simulink model "massbalancer"  (R2024a)
settings: Solver=VariableStepAuto  StartTime=0.0  StopTime=inf  RelTol=1e-3
libraries: matrix_library x36, sharedutil x2, sharedtransform x2, dspinverses x1, aerolibutil x1
(part 2 of 3)

== system massbalancer/Wdot b/I_r/Subsystem3 ==
  In1 : Inport
  Reshape : Reshape  OutputDimensionality=Column vector (2-D)  OutputDimensions=[1,3]
  Selector : Selector  InputPortWidth=9  IndexOptions=Index vector (dialog)  Indices=[1]  OutputSizes=1
  Selector1 : Selector  InputPortWidth=9  IndexOptions=Index vector (dialog)  Indices=[2]  OutputSizes=1
  Selector2 : Selector  InputPortWidth=9  IndexOptions=Index vector (dialog)  Indices=[3]  OutputSizes=1
  Selector3 : Selector  InputPortWidth=9  IndexOptions=Index vector (dialog)  Indices=[4]  OutputSizes=1
  Selector4 : Selector  InputPortWidth=9  IndexOptions=Index vector (dialog)  Indices=[5]  OutputSizes=1
  Selector5 : Selector  InputPortWidth=9  IndexOptions=Index vector (dialog)  Indices=[6]  OutputSizes=1
  Selector6 : Selector  InputPortWidth=9  IndexOptions=Index vector (dialog)  Indices=[7]  OutputSizes=1
  Selector7 : Selector  InputPortWidth=9  IndexOptions=Index vector (dialog)  Indices=[8]  OutputSizes=1
  Selector8 : Selector  InputPortWidth=9  IndexOptions=Index vector (dialog)  Indices=[9]  OutputSizes=1
  Vector Concatenate : Concatenate  NumInputs=3  Mode=Multidimensional array
  Vector Concatenate1 : Concatenate  NumInputs=3  Mode=Multidimensional array
  Vector Concatenate2 : Concatenate  NumInputs=3  Mode=Multidimensional array
  Out1 : Outport
  Out2 : Outport  Port=2
  Out3 : Outport  Port=3
  wires:
  Selector2/1 -> Vector Concatenate/3
  Vector Concatenate/1 -> Out1/1
  Selector8/1 -> Vector Concatenate2/3
  Selector4/1 -> Vector Concatenate1/2
  Selector6/1 -> Vector Concatenate2/1
  In1/1 -> Reshape/1
  Reshape/1 -> Selector8/1, Selector7/1, Selector6/1, Selector5/1, Selector4/1, Selector3/1, Selector2/1, Selector1/1, Selector/1
  Selector/1 -> Vector Concatenate/1
  Selector5/1 -> Vector Concatenate1/3
  Selector7/1 -> Vector Concatenate2/2
  Vector Concatenate2/1 -> Out3/1
  Vector Concatenate1/1 -> Out2/1
  Selector1/1 -> Vector Concatenate/2
  Selector3/1 -> Vector Concatenate1/1

== system massbalancer/Wdot b/I_r/Subsystem4 ==
  In1 : Inport
  Reshape : Reshape  OutputDimensionality=Column vector (2-D)  OutputDimensions=[1,3]
  Selector : Selector  InputPortWidth=9  IndexOptions=Index vector (dialog)  Indices=[1]  OutputSizes=1
  Selector1 : Selector  InputPortWidth=9  IndexOptions=Index vector (dialog)  Indices=[2]  OutputSizes=1
  Selector2 : Selector  InputPortWidth=9  IndexOptions=Index vector (dialog)  Indices=[3]  OutputSizes=1
  Selector3 : Selector  InputPortWidth=9  IndexOptions=Index vector (dialog)  Indices=[4]  OutputSizes=1
  Selector4 : Selector  InputPortWidth=9  IndexOptions=Index vector (dialog)  Indices=[5]  OutputSizes=1
  Selector5 : Selector  InputPortWidth=9  IndexOptions=Index vector (dialog)  Indices=[6]  OutputSizes=1
  Selector6 : Selector  InputPortWidth=9  IndexOptions=Index vector (dialog)  Indices=[7]  OutputSizes=1
  Selector7 : Selector  InputPortWidth=9  IndexOptions=Index vector (dialog)  Indices=[8]  OutputSizes=1
  Selector8 : Selector  InputPortWidth=9  IndexOptions=Index vector (dialog)  Indices=[9]  OutputSizes=1
  Vector Concatenate : Concatenate  NumInputs=3  Mode=Multidimensional array
  Vector Concatenate1 : Concatenate  NumInputs=3  Mode=Multidimensional array
  Vector Concatenate2 : Concatenate  NumInputs=3  Mode=Multidimensional array
  Out1 : Outport
  Out2 : Outport  Port=2
  Out3 : Outport  Port=3
  wires:
  Selector3/1 -> Vector Concatenate1/1
  Selector1/1 -> Vector Concatenate/2
  Vector Concatenate1/1 -> Out2/1
  Vector Concatenate2/1 -> Out3/1
  Selector7/1 -> Vector Concatenate2/2
  Selector5/1 -> Vector Concatenate1/3
  Selector/1 -> Vector Concatenate/1
  Reshape/1 -> Selector/1, Selector1/1, Selector2/1, Selector3/1, Selector4/1, Selector5/1, Selector6/1, Selector7/1, Selector8/1
  In1/1 -> Reshape/1
  Selector6/1 -> Vector Concatenate2/1
  Selector4/1 -> Vector Concatenate1/2
  Selector8/1 -> Vector Concatenate2/3
  Vector Concatenate/1 -> Out1/1
  Selector2/1 -> Vector Concatenate/3

== system massbalancer/Subsystem1/Subsystem1/Subsystem/Enabled Subsystem ==
  In1 : Inport
  Enable : EnablePort
  Out1 : Outport
  wires:
  In1/1 -> Out1/1

== system massbalancer/Subsystem1/Subsystem1/Subsystem1/Enabled Subsystem ==
  In1 : Inport
  Enable : EnablePort
  Out1 : Outport
  wires:
  In1/1 -> Out1/1

== system massbalancer/Subsystem1/Subsystem1/Subsystem2/Enabled Subsystem ==
  In1 : Inport
  Enable : EnablePort
  Out1 : Outport
  wires:
  In1/1 -> Out1/1

== system massbalancer/Subsystem1/Subsystem2/Subsystem/Enabled Subsystem ==
  In1 : Inport
  Enable : EnablePort
  Out1 : Outport
  wires:
  In1/1 -> Out1/1

== system massbalancer/Subsystem1/Subsystem2/Subsystem1/Enabled Subsystem ==
  In1 : Inport
  Enable : EnablePort
  Out1 : Outport
  wires:
  In1/1 -> Out1/1

== system massbalancer/Subsystem1/Subsystem2/Subsystem2/Enabled Subsystem ==
  In1 : Inport
  Enable : EnablePort
  Out1 : Outport
  wires:
  In1/1 -> Out1/1

== system massbalancer/Subsystem1/Subsystem3/Subsystem/Enabled Subsystem ==
  In1 : Inport
  Enable : EnablePort
  Out1 : Outport
  wires:
  In1/1 -> Out1/1

== system massbalancer/Subsystem1/Subsystem3/Subsystem1/Enabled Subsystem ==
  In1 : Inport
  Enable : EnablePort
  Out1 : Outport
  wires:
  In1/1 -> Out1/1

== system massbalancer/Subsystem1/Subsystem3/Subsystem2/Enabled Subsystem ==
  In1 : Inport
  Enable : EnablePort
  Out1 : Outport
  wires:
  In1/1 -> Out1/1

== system massbalancer/TNet/Subsystem1/R_I/Subsystem3 ==
  In1 : Inport
  Reshape : Reshape  OutputDimensionality=Column vector (2-D)  OutputDimensions=[1,3]
  Selector : Selector  InputPortWidth=9  IndexOptions=Index vector (dialog)  Indices=[1]  OutputSizes=1
  Selector1 : Selector  InputPortWidth=9  IndexOptions=Index vector (dialog)  Indices=[2]  OutputSizes=1
  Selector2 : Selector  InputPortWidth=9  IndexOptions=Index vector (dialog)  Indices=[3]  OutputSizes=1
  Selector3 : Selector  InputPortWidth=9  IndexOptions=Index vector (dialog)  Indices=[4]  OutputSizes=1
  Selector4 : Selector  InputPortWidth=9  IndexOptions=Index vector (dialog)  Indices=[5]  OutputSizes=1
  Selector5 : Selector  InputPortWidth=9  IndexOptions=Index vector (dialog)  Indices=[6]  OutputSizes=1
  Selector6 : Selector  InputPortWidth=9  IndexOptions=Index vector (dialog)  Indices=[7]  OutputSizes=1
  Selector7 : Selector  InputPortWidth=9  IndexOptions=Index vector (dialog)  Indices=[8]  OutputSizes=1
  Selector8 : Selector  InputPortWidth=9  IndexOptions=Index vector (dialog)  Indices=[9]  OutputSizes=1
  Vector Concatenate : Concatenate  NumInputs=3  Mode=Multidimensional array
  Vector Concatenate1 : Concatenate  NumInputs=3  Mode=Multidimensional array
  Vector Concatenate2 : Concatenate  NumInputs=3  Mode=Multidimensional array
  Out1 : Outport
  Out2 : Outport  Port=2
  Out3 : Outport  Port=3
  wires:
  Selector2/1 -> Vector Concatenate/3
  Vector Concatenate/1 -> Out1/1
  Selector8/1 -> Vector Concatenate2/3
  Selector4/1 -> Vector Concatenate1/2
  Selector6/1 -> Vector Concatenate2/1
  In1/1 -> Reshape/1
  Reshape/1 -> Selector8/1, Selector7/1, Selector6/1, Selector5/1, Selector4/1, Selector3/1, Selector2/1, Selector1/1, Selector/1
  Selector/1 -> Vector Concatenate/1
  Selector5/1 -> Vector Concatenate1/3
  Selector7/1 -> Vector Concatenate2/2
  Vector Concatenate2/1 -> Out3/1
  Vector Concatenate1/1 -> Out2/1
  Selector1/1 -> Vector Concatenate/2
  Selector3/1 -> Vector Concatenate1/1

== system massbalancer/TNet/Subsystem1/R_I/Subsystem4 ==
  In1 : Inport
  Reshape : Reshape  OutputDimensionality=Column vector (2-D)  OutputDimensions=[1,3]
  Selector : Selector  InputPortWidth=9  IndexOptions=Index vector (dialog)  Indices=[1]  OutputSizes=1
  Selector1 : Selector  InputPortWidth=9  IndexOptions=Index vector (dialog)  Indices=[2]  OutputSizes=1
  Selector2 : Selector  InputPortWidth=9  IndexOptions=Index vector (dialog)  Indices=[3]  OutputSizes=1
  Selector3 : Selector  InputPortWidth=9  IndexOptions=Index vector (dialog)  Indices=[4]  OutputSizes=1
  Selector4 : Selector  InputPortWidth=9  IndexOptions=Index vector (dialog)  Indices=[5]  OutputSizes=1
  Selector5 : Selector  InputPortWidth=9  IndexOptions=Index vector (dialog)  Indices=[6]  OutputSizes=1
  Selector6 : Selector  InputPortWidth=9  IndexOptions=Index vector (dialog)  Indices=[7]  OutputSizes=1
  Selector7 : Selector  InputPortWidth=9  IndexOptions=Index vector (dialog)  Indices=[8]  OutputSizes=1
  Selector8 : Selector  InputPortWidth=9  IndexOptions=Index vector (dialog)  Indices=[9]  OutputSizes=1
  Vector Concatenate : Concatenate  NumInputs=3  Mode=Multidimensional array
  Vector Concatenate1 : Concatenate  NumInputs=3  Mode=Multidimensional array
  Vector Concatenate2 : Concatenate  NumInputs=3  Mode=Multidimensional array
  Out1 : Outport
  Out2 : Outport  Port=2
  Out3 : Outport  Port=3
  wires:
  Selector3/1 -> Vector Concatenate1/1
  Selector1/1 -> Vector Concatenate/2
  Vector Concatenate1/1 -> Out2/1
  Vector Concatenate2/1 -> Out3/1
  Selector7/1 -> Vector Concatenate2/2
  Selector5/1 -> Vector Concatenate1/3
  Selector/1 -> Vector Concatenate/1
  Reshape/1 -> Selector/1, Selector1/1, Selector2/1, Selector3/1, Selector4/1, Selector5/1, Selector6/1, Selector7/1, Selector8/1
  In1/1 -> Reshape/1
  Selector6/1 -> Vector Concatenate2/1
  Selector4/1 -> Vector Concatenate1/2
  Selector8/1 -> Vector Concatenate2/3
  Vector Concatenate/1 -> Out1/1
  Selector2/1 -> Vector Concatenate/3

== system massbalancer/TNet/Subsystem1/Tbalances Init T Gravity /Fgravity ==
  Display : Display
  Matrix Multiply : Product  Multiplication=Matrix(*)
  Q(q) rotational form of quaternio : Subsystem
  Out1 : Outport
  wires:
  Q(q) rotational form of quaternio/1(Out1) -> Matrix Multiply/1
  [G] -> Matrix Multiply/2
  [q] -> Q(q) rotational form of quaternio/1(Q_input)
  Matrix Multiply/1 -> Display/1, Out1/1

== system massbalancer/TNet/Subsystem1/Tbalances Init T Gravity /Subsystem ==
  Output : Outport
  wires:
  [M_r] -> Output/1

== system massbalancer/TNet/Subsystem1/Term 1/R_I ==
  In1 : Inport
  Add : Sum
  Displacment D : Constant  Value=[0.05;-0.03;0.02]  VectorParams1D=off
  Matrix Concatenate1 : Concatenate  NumInputs=3  Mode=Multidimensional array  ConcatenateDimension=2
  Product : Product
  Product1 : Product
  Product2 : Product
  S value : Constant  Value=|
      | [ 0.9535,  0.2760,  0.0953;
      |       0.0953,  0.9206,  0.2859;
      |       0.2859,  0.2760,  0.9535 ]
  Selector : Selector  InputPortWidth=3  IndexOptions=Index vector (dialog)  Indices=[1]  OutputSizes=1
  Selector1 : Selector  InputPortWidth=3  IndexOptions=Index vector (dialog)  Indices=[2]  OutputSizes=1
  Selector2 : Selector  InputPortWidth=3  IndexOptions=Index vector (dialog)  Indices=[3]  OutputSizes=1
  Subsystem3 : Subsystem
  Subsystem4 : Subsystem
  Sum1 : Sum  Inputs=|++
  Sum2 : Sum  Inputs=|++
  R_0 : Outport
  wires:
  Subsystem4/1(Out1) -> Add/1
  Product1/1 -> Sum1/1
  Selector1/1 -> Product1/1
  Selector/1 -> Product/1
  Subsystem3/2(Out2) -> Product1/2
  Selector2/1 -> Product2/1
  Subsystem4/2(Out2) -> Sum1/2
  Displacment D/1 -> Selector/1, Selector1/1, Selector2/1
  Subsystem4/3(Out3) -> Sum2/2
  Product/1 -> Add/2
  Subsystem3/1(Out1) -> Product/2
  S value/1 -> Subsystem3/1(In1)
  Subsystem3/3(Out3) -> Product2/2
  Product2/1 -> Sum2/1
  In1/1 -> Subsystem4/1(In1)
  Add/1 -> Matrix Concatenate1/1
  Sum1/1 -> Matrix Concatenate1/2
  Sum2/1 -> Matrix Concatenate1/3
  Matrix Concatenate1/1 -> R_0/1

== system massbalancer/TNet/Subsystem1/Term 1/Subsystem1 ==
  R_0 : Inport
  Reshape : Reshape  OutputDimensionality=Column vector (2-D)  OutputDimensions=[1,3]
  Selector : Selector  InputPortWidth=9  IndexOptions=Index vector (dialog)  Indices=[1]  OutputSizes=1
  Selector1 : Selector  InputPortWidth=9  IndexOptions=Index vector (dialog)  Indices=[2]  OutputSizes=1
  Selector2 : Selector  InputPortWidth=9  IndexOptions=Index vector (dialog)  Indices=[3]  OutputSizes=1
  Selector3 : Selector  InputPortWidth=9  IndexOptions=Index vector (dialog)  Indices=[4]  OutputSizes=1
  Selector4 : Selector  InputPortWidth=9  IndexOptions=Index vector (dialog)  Indices=[5]  OutputSizes=1
  Selector5 : Selector  InputPortWidth=9  IndexOptions=Index vector (dialog)  Indices=[6]  OutputSizes=1
  Selector6 : Selector  InputPortWidth=9  IndexOptions=Index vector (dialog)  Indices=[7]  OutputSizes=1
  Selector7 : Selector  InputPortWidth=9  IndexOptions=Index vector (dialog)  Indices=[8]  OutputSizes=1
  Selector8 : Selector  InputPortWidth=9  IndexOptions=Index vector (dialog)  Indices=[9]  OutputSizes=1
  Vector Concatenate : Concatenate  NumInputs=3  Mode=Multidimensional array
  Vector Concatenate1 : Concatenate  NumInputs=3  Mode=Multidimensional array
  Vector Concatenate2 : Concatenate  NumInputs=3  Mode=Multidimensional array
  Out1 : Outport
  Out2 : Outport  Port=2
  Out3 : Outport  Port=3
  wires:
  Selector3/1 -> Vector Concatenate1/1
  Selector1/1 -> Vector Concatenate/2
  Vector Concatenate1/1 -> Out2/1
  Vector Concatenate2/1 -> Out3/1
  Selector7/1 -> Vector Concatenate2/2
  Selector5/1 -> Vector Concatenate1/3
  Selector/1 -> Vector Concatenate/1
  Reshape/1 -> Selector/1, Selector1/1, Selector2/1, Selector3/1, Selector4/1, Selector5/1, Selector6/1, Selector7/1, Selector8/1
  R_0/1 -> Reshape/1
  Selector6/1 -> Vector Concatenate2/1
  Selector4/1 -> Vector Concatenate1/2
  Selector8/1 -> Vector Concatenate2/3
  Vector Concatenate/1 -> Out1/1
  Selector2/1 -> Vector Concatenate/3

== system massbalancer/TNet/Subsystem1/Term 1/Subsystem3 ==
  R_0 : Inport
  Reshape : Reshape  OutputDimensionality=Column vector (2-D)  OutputDimensions=[1,3]
  Selector : Selector  InputPortWidth=9  IndexOptions=Index vector (dialog)  Indices=[1]  OutputSizes=1
  Selector1 : Selector  InputPortWidth=9  IndexOptions=Index vector (dialog)  Indices=[2]  OutputSizes=1
  Selector2 : Selector  InputPortWidth=9  IndexOptions=Index vector (dialog)  Indices=[3]  OutputSizes=1
  Selector3 : Selector  InputPortWidth=9  IndexOptions=Index vector (dialog)  Indices=[4]  OutputSizes=1
  Selector4 : Selector  InputPortWidth=9  IndexOptions=Index vector (dialog)  Indices=[5]  OutputSizes=1
  Selector5 : Selector  InputPortWidth=9  IndexOptions=Index vector (dialog)  Indices=[6]  OutputSizes=1
  Selector6 : Selector  InputPortWidth=9  IndexOptions=Index vector (dialog)  Indices=[7]  OutputSizes=1
  Selector7 : Selector  InputPortWidth=9  IndexOptions=Index vector (dialog)  Indices=[8]  OutputSizes=1
  Selector8 : Selector  InputPortWidth=9  IndexOptions=Index vector (dialog)  Indices=[9]  OutputSizes=1
  Vector Concatenate : Concatenate  NumInputs=3  Mode=Multidimensional array
  Vector Concatenate1 : Concatenate  NumInputs=3  Mode=Multidimensional array
  Vector Concatenate2 : Concatenate  NumInputs=3  Mode=Multidimensional array
  Out1 : Outport
  Out2 : Outport  Port=2
  Out3 : Outport  Port=3
  wires:
  Selector2/1 -> Vector Concatenate/3
  Vector Concatenate/1 -> Out1/1
  Selector8/1 -> Vector Concatenate2/3
  Selector4/1 -> Vector Concatenate1/2
  Selector6/1 -> Vector Concatenate2/1
  R_0/1 -> Reshape/1
  Reshape/1 -> Selector8/1, Selector7/1, Selector6/1, Selector5/1, Selector4/1, Selector3/1, Selector2/1, Selector1/1, Selector/1
  Selector/1 -> Vector Concatenate/1
  Selector5/1 -> Vector Concatenate1/3
  Selector7/1 -> Vector Concatenate2/2
  Vector Concatenate2/1 -> Out3/1
  Vector Concatenate1/1 -> Out2/1
  Selector1/1 -> Vector Concatenate/2
  Selector3/1 -> Vector Concatenate1/1

== system massbalancer/TNet/Subsystem1/Term 1/X ==
  R-0 : Inport
  dd : Inport  Port=2
  s : Inport  Port=3
  Wb : Inport  Port=4
  Cross Product : matrix_library/Cross Product
  Cross Product1 : matrix_library/Cross Product
  Product : Product
  y : Outport
  wires:
  Cross Product1/1 -> Cross Product/2
  s/1 -> Product/2
  dd/1 -> Product/1
  Wb/1 -> Cross Product1/1
  Cross Product/1 -> y/1
  Product/1 -> Cross Product/1
  R-0/1 -> Cross Product1/2

== system massbalancer/TNet/Subsystem1/Term 1/Y ==
  R0 : Inport
  ddot : Inport  Port=2
  s : Inport  Port=3
  Wb : Inport  Port=4
  Cross Product : matrix_library/Cross Product
  Cross Product1 : matrix_library/Cross Product
  Product : Product
  y : Outport
  wires:
  Wb/1 -> Cross Product/1
  Cross Product/1 -> Cross Product1/2
  Product/1 -> Cross Product1/1
  Cross Product1/1 -> y/1
  ddot/1 -> Product/1
  s/1 -> Product/2
  R0/1 -> Cross Product/2

== system massbalancer/TNet/Subsystem1/Term 1/Z ==
  ddot : Inport
  R0 : Inport  Port=2
  s : Inport  Port=3
  Wb : Inport  Port=4
  Cross Product : matrix_library/Cross Product
  Cross Product1 : matrix_library/Cross Product
  Product : Product
  y : Outport
  wires:
  ddot/1 -> Product/2
  Cross Product1/1 -> y/1
  Product/1 -> Cross Product1/1
  Cross Product/1 -> Cross Product1/2
  s/1 -> Product/1
  Wb/1 -> Cross Product/1
  R0/1 -> Cross Product/2

== system massbalancer/TNet/Subsystem1/Term2/R_I ==
  In1 : Inport
  Add : Sum
  Displacment D : Constant  Value=[0.05;-0.03;0.02]  VectorParams1D=off
  Matrix Concatenate1 : Concatenate  NumInputs=3  Mode=Multidimensional array  ConcatenateDimension=2
  Product : Product
  Product1 : Product
  Product2 : Product
  S value : Constant  Value=|
      | [ 0.9535,  0.2760,  0.0953;
      |       0.0953,  0.9206,  0.2859;
      |       0.2859,  0.2760,  0.9535 ]
  Selector : Selector  InputPortWidth=3  IndexOptions=Index vector (dialog)  Indices=[1]  OutputSizes=1
  Selector1 : Selector  InputPortWidth=3  IndexOptions=Index vector (dialog)  Indices=[2]  OutputSizes=1
  Selector2 : Selector  InputPortWidth=3  IndexOptions=Index vector (dialog)  Indices=[3]  OutputSizes=1
  Subsystem3 : Subsystem
  Subsystem4 : Subsystem
  Sum1 : Sum  Inputs=|++
  Sum2 : Sum  Inputs=|++
  R_0 : Outport
  wires:
  Subsystem4/1(Out1) -> Add/1
  Product1/1 -> Sum1/1
  Selector1/1 -> Product1/1
  Selector/1 -> Product/1
  Subsystem3/2(Out2) -> Product1/2
  Selector2/1 -> Product2/1
  Subsystem4/2(Out2) -> Sum1/2
  Displacment D/1 -> Selector/1, Selector1/1, Selector2/1
  Subsystem4/3(Out3) -> Sum2/2
  Product/1 -> Add/2
  Subsystem3/1(Out1) -> Product/2
  S value/1 -> Subsystem3/1(In1)
  Subsystem3/3(Out3) -> Product2/2
  Product2/1 -> Sum2/1
  In1/1 -> Subsystem4/1(In1)
  Add/1 -> Matrix Concatenate1/1
  Sum1/1 -> Matrix Concatenate1/2
  Sum2/1 -> Matrix Concatenate1/3
  Matrix Concatenate1/1 -> R_0/1

== system massbalancer/TNet/Subsystem1/Term2/Subsystem1 ==
  R_0 : Inport
  Reshape : Reshape  OutputDimensionality=Column vector (2-D)  OutputDimensions=[1,3]
  Selector : Selector  InputPortWidth=9  IndexOptions=Index vector (dialog)  Indices=[1]  OutputSizes=1
  Selector1 : Selector  InputPortWidth=9  IndexOptions=Index vector (dialog)  Indices=[2]  OutputSizes=1
  Selector2 : Selector  InputPortWidth=9  IndexOptions=Index vector (dialog)  Indices=[3]  OutputSizes=1
  Selector3 : Selector  InputPortWidth=9  IndexOptions=Index vector (dialog)  Indices=[4]  OutputSizes=1
  Selector4 : Selector  InputPortWidth=9  IndexOptions=Index vector (dialog)  Indices=[5]  OutputSizes=1
  Selector5 : Selector  InputPortWidth=9  IndexOptions=Index vector (dialog)  Indices=[6]  OutputSizes=1
  Selector6 : Selector  InputPortWidth=9  IndexOptions=Index vector (dialog)  Indices=[7]  OutputSizes=1
  Selector7 : Selector  InputPortWidth=9  IndexOptions=Index vector (dialog)  Indices=[8]  OutputSizes=1
  Selector8 : Selector  InputPortWidth=9  IndexOptions=Index vector (dialog)  Indices=[9]  OutputSizes=1
  Vector Concatenate : Concatenate  NumInputs=3  Mode=Multidimensional array
  Vector Concatenate1 : Concatenate  NumInputs=3  Mode=Multidimensional array
  Vector Concatenate2 : Concatenate  NumInputs=3  Mode=Multidimensional array
  Out1 : Outport
  Out2 : Outport  Port=2
  Out3 : Outport  Port=3
  wires:
  Selector3/1 -> Vector Concatenate1/1
  Selector1/1 -> Vector Concatenate/2
  Vector Concatenate1/1 -> Out2/1
  Vector Concatenate2/1 -> Out3/1
  Selector7/1 -> Vector Concatenate2/2
  Selector5/1 -> Vector Concatenate1/3
  Selector/1 -> Vector Concatenate/1
  Reshape/1 -> Selector/1, Selector1/1, Selector2/1, Selector3/1, Selector4/1, Selector5/1, Selector6/1, Selector7/1, Selector8/1
  R_0/1 -> Reshape/1
  Selector6/1 -> Vector Concatenate2/1
  Selector4/1 -> Vector Concatenate1/2
  Selector8/1 -> Vector Concatenate2/3
  Vector Concatenate/1 -> Out1/1
  Selector2/1 -> Vector Concatenate/3

== system massbalancer/TNet/Subsystem1/Term2/Subsystem3 ==
  R_0 : Inport
  Reshape : Reshape  OutputDimensionality=Column vector (2-D)  OutputDimensions=[1,3]
  Selector : Selector  InputPortWidth=9  IndexOptions=Index vector (dialog)  Indices=[1]  OutputSizes=1
  Selector1 : Selector  InputPortWidth=9  IndexOptions=Index vector (dialog)  Indices=[2]  OutputSizes=1
  Selector2 : Selector  InputPortWidth=9  IndexOptions=Index vector (dialog)  Indices=[3]  OutputSizes=1
  Selector3 : Selector  InputPortWidth=9  IndexOptions=Index vector (dialog)  Indices=[4]  OutputSizes=1
  Selector4 : Selector  InputPortWidth=9  IndexOptions=Index vector (dialog)  Indices=[5]  OutputSizes=1
  Selector5 : Selector  InputPortWidth=9  IndexOptions=Index vector (dialog)  Indices=[6]  OutputSizes=1
  Selector6 : Selector  InputPortWidth=9  IndexOptions=Index vector (dialog)  Indices=[7]  OutputSizes=1
  Selector7 : Selector  InputPortWidth=9  IndexOptions=Index vector (dialog)  Indices=[8]  OutputSizes=1
  Selector8 : Selector  InputPortWidth=9  IndexOptions=Index vector (dialog)  Indices=[9]  OutputSizes=1
  Vector Concatenate : Concatenate  NumInputs=3  Mode=Multidimensional array
  Vector Concatenate1 : Concatenate  NumInputs=3  Mode=Multidimensional array
  Vector Concatenate2 : Concatenate  NumInputs=3  Mode=Multidimensional array
  Out1 : Outport
  Out2 : Outport  Port=2
  Out3 : Outport  Port=3
  wires:
  Selector2/1 -> Vector Concatenate/3
  Vector Concatenate/1 -> Out1/1
  Selector8/1 -> Vector Concatenate2/3
  Selector4/1 -> Vector Concatenate1/2
  Selector6/1 -> Vector Concatenate2/1
  R_0/1 -> Reshape/1
  Reshape/1 -> Selector8/1, Selector7/1, Selector6/1, Selector5/1, Selector4/1, Selector3/1, Selector2/1, Selector1/1, Selector/1
  Selector/1 -> Vector Concatenate/1
  Selector5/1 -> Vector Concatenate1/3
  Selector7/1 -> Vector Concatenate2/2
  Vector Concatenate2/1 -> Out3/1
  Vector Concatenate1/1 -> Out2/1
  Selector1/1 -> Vector Concatenate/2
  Selector3/1 -> Vector Concatenate1/1

== system massbalancer/TNet/Subsystem1/Term2/X ==
  R-0 : Inport
  Ddot : Inport  Port=2
  s : Inport  Port=3
  Wb : Inport  Port=4
  Cross Product : matrix_library/Cross Product
  Cross Product1 : matrix_library/Cross Product
  Display{,1..5} (6 alike) : Display
  Product : Product
  Output : Outport
  wires:
  Cross Product1/1 -> Display/1, Output/1
  R-0/1 -> Cross Product1/1
  Product/1 -> Cross Product/2, Display1/1
  s/1 -> Display4/1, Product/2
  Ddot/1 -> Display5/1, Product/1
  Wb/1 -> Cross Product/1, Display3/1
  Cross Product/1 -> Display2/1, Cross Product1/2

== system massbalancer/TNet/Subsystem1/Term2/Y ==
  R0 : Inport
  ddot : Inport  Port=2
  s : Inport  Port=3
  Wb : Inport  Port=4
  Cross Product : matrix_library/Cross Product
  Cross Product1 : matrix_library/Cross Product
  Product : Product
  Output : Outport
  wires:
  s/1 -> Product/1
  Product/1 -> Cross Product/2
  R0/1 -> Cross Product1/1
  Cross Product/1 -> Cross Product1/2
  ddot/1 -> Product/2
  Wb/1 -> Cross Product/1
  Cross Product1/1 -> Output/1

== system massbalancer/TNet/Subsystem1/Term2/Z ==
  ddot : Inport
  R0 : Inport  Port=2
  s : Inport  Port=3
  Wb : Inport  Port=4
  Cross Product : matrix_library/Cross Product
  Cross Product1 : matrix_library/Cross Product
  Product : Product
  Output1 : Outport
  wires:
  s/1 -> Product/1
  Product/1 -> Cross Product/2
  R0/1 -> Cross Product1/1
  Cross Product/1 -> Cross Product1/2
  ddot/1 -> Product/2
  Wb/1 -> Cross Product/1
  Cross Product1/1 -> Output1/1

== system massbalancer/TNet/Subsystem1/Term3/Subsystem1 ==
  R_0 : Inport
  Reshape : Reshape  OutputDimensionality=Column vector (2-D)  OutputDimensions=[1,3]
  Selector : Selector  InputPortWidth=9  IndexOptions=Index vector (dialog)  Indices=[1]  OutputSizes=1
  Selector1 : Selector  InputPortWidth=9  IndexOptions=Index vector (dialog)  Indices=[2]  OutputSizes=1
  Selector2 : Selector  InputPortWidth=9  IndexOptions=Index vector (dialog)  Indices=[3]  OutputSizes=1
  Selector3 : Selector  InputPortWidth=9  IndexOptions=Index vector (dialog)  Indices=[4]  OutputSizes=1
  Selector4 : Selector  InputPortWidth=9  IndexOptions=Index vector (dialog)  Indices=[5]  OutputSizes=1
  Selector5 : Selector  InputPortWidth=9  IndexOptions=Index vector (dialog)  Indices=[6]  OutputSizes=1
  Selector6 : Selector  InputPortWidth=9  IndexOptions=Index vector (dialog)  Indices=[7]  OutputSizes=1
  Selector7 : Selector  InputPortWidth=9  IndexOptions=Index vector (dialog)  Indices=[8]  OutputSizes=1
  Selector8 : Selector  InputPortWidth=9  IndexOptions=Index vector (dialog)  Indices=[9]  OutputSizes=1
  Vector Concatenate : Concatenate  NumInputs=3  Mode=Multidimensional array
  Vector Concatenate1 : Concatenate  NumInputs=3  Mode=Multidimensional array
  Vector Concatenate2 : Concatenate  NumInputs=3  Mode=Multidimensional array
  Out1 : Outport
  Out2 : Outport  Port=2
  Out3 : Outport  Port=3
  wires:
  Selector3/1 -> Vector Concatenate1/1
  Selector1/1 -> Vector Concatenate/2
  Vector Concatenate1/1 -> Out2/1
  Vector Concatenate2/1 -> Out3/1
  Selector7/1 -> Vector Concatenate2/2
  Selector5/1 -> Vector Concatenate1/3
  Selector/1 -> Vector Concatenate/1
  Reshape/1 -> Selector/1, Selector1/1, Selector2/1, Selector3/1, Selector4/1, Selector5/1, Selector6/1, Selector7/1, Selector8/1
  R_0/1 -> Reshape/1
  Selector6/1 -> Vector Concatenate2/1
  Selector4/1 -> Vector Concatenate1/2
  Selector8/1 -> Vector Concatenate2/3
  Vector Concatenate/1 -> Out1/1
  Selector2/1 -> Vector Concatenate/3

== system massbalancer/TNet/Subsystem1/Term3/Subsystem3 ==
  R_0 : Inport
  Reshape : Reshape  OutputDimensionality=Column vector (2-D)  OutputDimensions=[1,3]
  Selector : Selector  InputPortWidth=9  IndexOptions=Index vector (dialog)  Indices=[1]  OutputSizes=1
  Selector1 : Selector  InputPortWidth=9  IndexOptions=Index vector (dialog)  Indices=[2]  OutputSizes=1
  Selector2 : Selector  InputPortWidth=9  IndexOptions=Index vector (dialog)  Indices=[3]  OutputSizes=1
  Selector3 : Selector  InputPortWidth=9  IndexOptions=Index vector (dialog)  Indices=[4]  OutputSizes=1
  Selector4 : Selector  InputPortWidth=9  IndexOptions=Index vector (dialog)  Indices=[5]  OutputSizes=1
  Selector5 : Selector  InputPortWidth=9  IndexOptions=Index vector (dialog)  Indices=[6]  OutputSizes=1
  Selector6 : Selector  InputPortWidth=9  IndexOptions=Index vector (dialog)  Indices=[7]  OutputSizes=1
  Selector7 : Selector  InputPortWidth=9  IndexOptions=Index vector (dialog)  Indices=[8]  OutputSizes=1
  Selector8 : Selector  InputPortWidth=9  IndexOptions=Index vector (dialog)  Indices=[9]  OutputSizes=1
  Vector Concatenate : Concatenate  NumInputs=3  Mode=Multidimensional array
  Vector Concatenate1 : Concatenate  NumInputs=3  Mode=Multidimensional array
  Vector Concatenate2 : Concatenate  NumInputs=3  Mode=Multidimensional array
  Out1 : Outport
  Out2 : Outport  Port=2
  Out3 : Outport  Port=3
  wires:
  Selector2/1 -> Vector Concatenate/3
  Vector Concatenate/1 -> Out1/1
  Selector8/1 -> Vector Concatenate2/3
  Selector4/1 -> Vector Concatenate1/2
  Selector6/1 -> Vector Concatenate2/1
  R_0/1 -> Reshape/1
  Reshape/1 -> Selector8/1, Selector7/1, Selector6/1, Selector5/1, Selector4/1, Selector3/1, Selector2/1, Selector1/1, Selector/1
  Selector/1 -> Vector Concatenate/1
  Selector5/1 -> Vector Concatenate1/3
  Selector7/1 -> Vector Concatenate2/2
  Vector Concatenate2/1 -> Out3/1
  Vector Concatenate1/1 -> Out2/1
  Selector1/1 -> Vector Concatenate/2
  Selector3/1 -> Vector Concatenate1/1

== system massbalancer/TNet/Subsystem1/Term3/X ==
  ddoubledot : Inport
  s : Inport  Port=2
  r : Inport  Port=3
  Cross Product : matrix_library/Cross Product
  Display : Display
  Display1 : Display
  Display2 : Display
  Product : Product
  y : Outport
  wires:
  Cross Product/1 -> y/1
  ddoubledot/1 -> Display2/1, Product/1
  Product/1 -> Display/1, Cross Product/2
  r/1 -> Cross Product/1
  s/1 -> Product/2, Display1/1

== system massbalancer/TNet/Subsystem1/Term3/Y ==
  ddoubledot : Inport
  s : Inport  Port=2
  r : Inport  Port=3
  Cross Product : matrix_library/Cross Product
  Display : Display
  Product : Product
  y : Outport
  wires:
  Cross Product/1 -> y/1
  ddoubledot/1 -> Product/1
  Product/1 -> Cross Product/2
  r/1 -> Display/1, Cross Product/1
  s/1 -> Product/2

== system massbalancer/TNet/Subsystem1/Term3/Z ==
  r : Inport
  s : Inport  Port=2
  ddoubledot : Inport  Port=3
  Cross Product : matrix_library/Cross Product
  Display : Display
  Display1 : Display
  Product : Product
  y : Outport
  wires:
  Cross Product/1 -> Display/1, y/1
  ddoubledot/1 -> Display1/1, Product/1
  s/1 -> Product/2
  Product/1 -> Cross Product/2
  r/1 -> Cross Product/1

== system massbalancer/TNet/TBalances/R_I/Subsystem3 ==
  In1 : Inport
  Reshape : Reshape  OutputDimensionality=Column vector (2-D)  OutputDimensions=[1,3]
  Selector : Selector  InputPortWidth=9  IndexOptions=Index vector (dialog)  Indices=[1]  OutputSizes=1
  Selector1 : Selector  InputPortWidth=9  IndexOptions=Index vector (dialog)  Indices=[2]  OutputSizes=1
  Selector2 : Selector  InputPortWidth=9  IndexOptions=Index vector (dialog)  Indices=[3]  OutputSizes=1
  Selector3 : Selector  InputPortWidth=9  IndexOptions=Index vector (dialog)  Indices=[4]  OutputSizes=1
  Selector4 : Selector  InputPortWidth=9  IndexOptions=Index vector (dialog)  Indices=[5]  OutputSizes=1
  Selector5 : Selector  InputPortWidth=9  IndexOptions=Index vector (dialog)  Indices=[6]  OutputSizes=1
  Selector6 : Selector  InputPortWidth=9  IndexOptions=Index vector (dialog)  Indices=[7]  OutputSizes=1
  Selector7 : Selector  InputPortWidth=9  IndexOptions=Index vector (dialog)  Indices=[8]  OutputSizes=1
  Selector8 : Selector  InputPortWidth=9  IndexOptions=Index vector (dialog)  Indices=[9]  OutputSizes=1
  Vector Concatenate : Concatenate  NumInputs=3  Mode=Multidimensional array
  Vector Concatenate1 : Concatenate  NumInputs=3  Mode=Multidimensional array
  Vector Concatenate2 : Concatenate  NumInputs=3  Mode=Multidimensional array
  Out1 : Outport
  Out2 : Outport  Port=2
  Out3 : Outport  Port=3
  wires:
  Selector2/1 -> Vector Concatenate/3
  Vector Concatenate/1 -> Out1/1
  Selector8/1 -> Vector Concatenate2/3
  Selector4/1 -> Vector Concatenate1/2
  Selector6/1 -> Vector Concatenate2/1
  In1/1 -> Reshape/1
  Reshape/1 -> Selector8/1, Selector7/1, Selector6/1, Selector5/1, Selector4/1, Selector3/1, Selector2/1, Selector1/1, Selector/1
  Selector/1 -> Vector Concatenate/1
  Selector5/1 -> Vector Concatenate1/3
  Selector7/1 -> Vector Concatenate2/2
  Vector Concatenate2/1 -> Out3/1
  Vector Concatenate1/1 -> Out2/1
  Selector1/1 -> Vector Concatenate/2
  Selector3/1 -> Vector Concatenate1/1

== system massbalancer/TNet/TBalances/R_I/Subsystem4 ==
  In1 : Inport
  Reshape : Reshape  OutputDimensionality=Column vector (2-D)  OutputDimensions=[1,3]
  Selector : Selector  InputPortWidth=9  IndexOptions=Index vector (dialog)  Indices=[1]  OutputSizes=1
  Selector1 : Selector  InputPortWidth=9  IndexOptions=Index vector (dialog)  Indices=[2]  OutputSizes=1
  Selector2 : Selector  InputPortWidth=9  IndexOptions=Index vector (dialog)  Indices=[3]  OutputSizes=1
  Selector3 : Selector  InputPortWidth=9  IndexOptions=Index vector (dialog)  Indices=[4]  OutputSizes=1
  Selector4 : Selector  InputPortWidth=9  IndexOptions=Index vector (dialog)  Indices=[5]  OutputSizes=1
  Selector5 : Selector  InputPortWidth=9  IndexOptions=Index vector (dialog)  Indices=[6]  OutputSizes=1
  Selector6 : Selector  InputPortWidth=9  IndexOptions=Index vector (dialog)  Indices=[7]  OutputSizes=1
  Selector7 : Selector  InputPortWidth=9  IndexOptions=Index vector (dialog)  Indices=[8]  OutputSizes=1
  Selector8 : Selector  InputPortWidth=9  IndexOptions=Index vector (dialog)  Indices=[9]  OutputSizes=1
  Vector Concatenate : Concatenate  NumInputs=3  Mode=Multidimensional array
  Vector Concatenate1 : Concatenate  NumInputs=3  Mode=Multidimensional array
  Vector Concatenate2 : Concatenate  NumInputs=3  Mode=Multidimensional array
  Out1 : Outport
  Out2 : Outport  Port=2
  Out3 : Outport  Port=3
  wires:
  Selector3/1 -> Vector Concatenate1/1
  Selector1/1 -> Vector Concatenate/2
  Vector Concatenate1/1 -> Out2/1
  Vector Concatenate2/1 -> Out3/1
  Selector7/1 -> Vector Concatenate2/2
  Selector5/1 -> Vector Concatenate1/3
  Selector/1 -> Vector Concatenate/1
  Reshape/1 -> Selector/1, Selector1/1, Selector2/1, Selector3/1, Selector4/1, Selector5/1, Selector6/1, Selector7/1, Selector8/1
  In1/1 -> Reshape/1
  Selector6/1 -> Vector Concatenate2/1
  Selector4/1 -> Vector Concatenate1/2
  Selector8/1 -> Vector Concatenate2/3
  Vector Concatenate/1 -> Out1/1
  Selector2/1 -> Vector Concatenate/3

== system massbalancer/TNet/TBalances/Term1/Subsystem1 ==
  R_0 : Inport
  Reshape : Reshape  OutputDimensionality=Column vector (2-D)  OutputDimensions=[1,3]
  Selector : Selector  InputPortWidth=9  IndexOptions=Index vector (dialog)  Indices=[1]  OutputSizes=1
  Selector1 : Selector  InputPortWidth=9  IndexOptions=Index vector (dialog)  Indices=[2]  OutputSizes=1
  Selector2 : Selector  InputPortWidth=9  IndexOptions=Index vector (dialog)  Indices=[3]  OutputSizes=1
  Selector3 : Selector  InputPortWidth=9  IndexOptions=Index vector (dialog)  Indices=[4]  OutputSizes=1
  Selector4 : Selector  InputPortWidth=9  IndexOptions=Index vector (dialog)  Indices=[5]  OutputSizes=1
  Selector5 : Selector  InputPortWidth=9  IndexOptions=Index vector (dialog)  Indices=[6]  OutputSizes=1
  Selector6 : Selector  InputPortWidth=9  IndexOptions=Index vector (dialog)  Indices=[7]  OutputSizes=1
  Selector7 : Selector  InputPortWidth=9  IndexOptions=Index vector (dialog)  Indices=[8]  OutputSizes=1
  Selector8 : Selector  InputPortWidth=9  IndexOptions=Index vector (dialog)  Indices=[9]  OutputSizes=1
  Vector Concatenate : Concatenate  NumInputs=3  Mode=Multidimensional array
  Vector Concatenate1 : Concatenate  NumInputs=3  Mode=Multidimensional array
  Vector Concatenate2 : Concatenate  NumInputs=3  Mode=Multidimensional array
  Out1 : Outport
  Out2 : Outport  Port=2
  Out3 : Outport  Port=3
  wires:
  Selector3/1 -> Vector Concatenate1/1
  Selector1/1 -> Vector Concatenate/2
  Vector Concatenate1/1 -> Out2/1
  Vector Concatenate2/1 -> Out3/1
  Selector7/1 -> Vector Concatenate2/2
  Selector5/1 -> Vector Concatenate1/3
  Selector/1 -> Vector Concatenate/1
  Reshape/1 -> Selector/1, Selector1/1, Selector2/1, Selector3/1, Selector4/1, Selector5/1, Selector6/1, Selector7/1, Selector8/1
  R_0/1 -> Reshape/1
  Selector6/1 -> Vector Concatenate2/1
  Selector4/1 -> Vector Concatenate1/2
  Selector8/1 -> Vector Concatenate2/3
  Vector Concatenate/1 -> Out1/1
  Selector2/1 -> Vector Concatenate/3

== system massbalancer/TNet/TBalances/Term1/Subsystem3 ==
  R_0 : Inport
  Reshape : Reshape  OutputDimensionality=Column vector (2-D)  OutputDimensions=[1,3]
  Selector : Selector  InputPortWidth=9  IndexOptions=Index vector (dialog)  Indices=[1]  OutputSizes=1
  Selector1 : Selector  InputPortWidth=9  IndexOptions=Index vector (dialog)  Indices=[2]  OutputSizes=1
  Selector2 : Selector  InputPortWidth=9  IndexOptions=Index vector (dialog)  Indices=[3]  OutputSizes=1
  Selector3 : Selector  InputPortWidth=9  IndexOptions=Index vector (dialog)  Indices=[4]  OutputSizes=1
  Selector4 : Selector  InputPortWidth=9  IndexOptions=Index vector (dialog)  Indices=[5]  OutputSizes=1
  Selector5 : Selector  InputPortWidth=9  IndexOptions=Index vector (dialog)  Indices=[6]  OutputSizes=1
  Selector6 : Selector  InputPortWidth=9  IndexOptions=Index vector (dialog)  Indices=[7]  OutputSizes=1
  Selector7 : Selector  InputPortWidth=9  IndexOptions=Index vector (dialog)  Indices=[8]  OutputSizes=1
  Selector8 : Selector  InputPortWidth=9  IndexOptions=Index vector (dialog)  Indices=[9]  OutputSizes=1
  Vector Concatenate : Concatenate  NumInputs=3  Mode=Multidimensional array
  Vector Concatenate1 : Concatenate  NumInputs=3  Mode=Multidimensional array
  Vector Concatenate2 : Concatenate  NumInputs=3  Mode=Multidimensional array
  Out1 : Outport
  Out2 : Outport  Port=2
  Out3 : Outport  Port=3
  wires:
  Selector2/1 -> Vector Concatenate/3
  Vector Concatenate/1 -> Out1/1
  Selector8/1 -> Vector Concatenate2/3
  Selector4/1 -> Vector Concatenate1/2
  Selector6/1 -> Vector Concatenate2/1
  R_0/1 -> Reshape/1
  Reshape/1 -> Selector8/1, Selector7/1, Selector6/1, Selector5/1, Selector4/1, Selector3/1, Selector2/1, Selector1/1, Selector/1
  Selector/1 -> Vector Concatenate/1
  Selector5/1 -> Vector Concatenate1/3
  Selector7/1 -> Vector Concatenate2/2
  Vector Concatenate2/1 -> Out3/1
  Vector Concatenate1/1 -> Out2/1
  Selector1/1 -> Vector Concatenate/2
  Selector3/1 -> Vector Concatenate1/1

== system massbalancer/TNet/TBalances/Term1/X ==
  R-0 : Inport
  dd : Inport  Port=2
  s : Inport  Port=3
  Wb : Inport  Port=4
  Cross Product : matrix_library/Cross Product
  Cross Product1 : matrix_library/Cross Product
  Display : Display
  Product : Product
  y : Outport
  wires:
  Product/1 -> Cross Product1/1
  Cross Product/1 -> Cross Product1/2
  Wb/1 -> Cross Product/1
  R-0/1 -> Cross Product/2
  Cross Product1/1 -> Display/1, y/1
  s/1 -> Product/2
  dd/1 -> Product/1

== system massbalancer/TNet/TBalances/Term1/Y ==
  R0 : Inport
  ddot : Inport  Port=2
  s : Inport  Port=3
  Wb : Inport  Port=4
  Cross Product : matrix_library/Cross Product
  Cross Product1 : matrix_library/Cross Product
  Display : Display
  Product : Product
  y : Outport
  wires:
  R0/1 -> Cross Product/2
  Wb/1 -> Cross Product/1
  s/1 -> Product/1
  Cross Product/1 -> Cross Product1/2
  Product/1 -> Cross Product1/1
  Cross Product1/1 -> Display/1, y/1
  ddot/1 -> Product/2

== system massbalancer/TNet/TBalances/Term1/Z ==
  ddot : Inport
  R0 : Inport  Port=2
  s : Inport  Port=3
  Wb : Inport  Port=4
  Cross Product : matrix_library/Cross Product
  Cross Product1 : matrix_library/Cross Product
  Product : Product
  y : Outport
  wires:
  ddot/1 -> Product/2
  Cross Product1/1 -> y/1
  Product/1 -> Cross Product1/1
  Cross Product/1 -> Cross Product1/2
  s/1 -> Product/1
  Wb/1 -> Cross Product/1
  R0/1 -> Cross Product/2

== system massbalancer/TNet/TBalances/Term2/Subsystem1 ==
  R_0 : Inport
  Reshape : Reshape  OutputDimensionality=Column vector (2-D)  OutputDimensions=[1,3]
  Selector : Selector  InputPortWidth=9  IndexOptions=Index vector (dialog)  Indices=[1]  OutputSizes=1
  Selector1 : Selector  InputPortWidth=9  IndexOptions=Index vector (dialog)  Indices=[2]  OutputSizes=1
  Selector2 : Selector  InputPortWidth=9  IndexOptions=Index vector (dialog)  Indices=[3]  OutputSizes=1
  Selector3 : Selector  InputPortWidth=9  IndexOptions=Index vector (dialog)  Indices=[4]  OutputSizes=1
  Selector4 : Selector  InputPortWidth=9  IndexOptions=Index vector (dialog)  Indices=[5]  OutputSizes=1
  Selector5 : Selector  InputPortWidth=9  IndexOptions=Index vector (dialog)  Indices=[6]  OutputSizes=1
  Selector6 : Selector  InputPortWidth=9  IndexOptions=Index vector (dialog)  Indices=[7]  OutputSizes=1
  Selector7 : Selector  InputPortWidth=9  IndexOptions=Index vector (dialog)  Indices=[8]  OutputSizes=1
  Selector8 : Selector  InputPortWidth=9  IndexOptions=Index vector (dialog)  Indices=[9]  OutputSizes=1
  Vector Concatenate : Concatenate  NumInputs=3  Mode=Multidimensional array
  Vector Concatenate1 : Concatenate  NumInputs=3  Mode=Multidimensional array
  Vector Concatenate2 : Concatenate  NumInputs=3  Mode=Multidimensional array
  Out1 : Outport
  Out2 : Outport  Port=2
  Out3 : Outport  Port=3
  wires:
  Selector3/1 -> Vector Concatenate1/1
  Selector1/1 -> Vector Concatenate/2
  Vector Concatenate1/1 -> Out2/1
  Vector Concatenate2/1 -> Out3/1
  Selector7/1 -> Vector Concatenate2/2
  Selector5/1 -> Vector Concatenate1/3
  Selector/1 -> Vector Concatenate/1
  Reshape/1 -> Selector/1, Selector1/1, Selector2/1, Selector3/1, Selector4/1, Selector5/1, Selector6/1, Selector7/1, Selector8/1
  R_0/1 -> Reshape/1
  Selector6/1 -> Vector Concatenate2/1
  Selector4/1 -> Vector Concatenate1/2
  Selector8/1 -> Vector Concatenate2/3
  Vector Concatenate/1 -> Out1/1
  Selector2/1 -> Vector Concatenate/3

== system massbalancer/TNet/TBalances/Term2/Subsystem3 ==
  R_0 : Inport
  Reshape : Reshape  OutputDimensionality=Column vector (2-D)  OutputDimensions=[1,3]
  Selector : Selector  InputPortWidth=9  IndexOptions=Index vector (dialog)  Indices=[1]  OutputSizes=1
  Selector1 : Selector  InputPortWidth=9  IndexOptions=Index vector (dialog)  Indices=[2]  OutputSizes=1
  Selector2 : Selector  InputPortWidth=9  IndexOptions=Index vector (dialog)  Indices=[3]  OutputSizes=1
  Selector3 : Selector  InputPortWidth=9  IndexOptions=Index vector (dialog)  Indices=[4]  OutputSizes=1
  Selector4 : Selector  InputPortWidth=9  IndexOptions=Index vector (dialog)  Indices=[5]  OutputSizes=1
  Selector5 : Selector  InputPortWidth=9  IndexOptions=Index vector (dialog)  Indices=[6]  OutputSizes=1
  Selector6 : Selector  InputPortWidth=9  IndexOptions=Index vector (dialog)  Indices=[7]  OutputSizes=1
  Selector7 : Selector  InputPortWidth=9  IndexOptions=Index vector (dialog)  Indices=[8]  OutputSizes=1
  Selector8 : Selector  InputPortWidth=9  IndexOptions=Index vector (dialog)  Indices=[9]  OutputSizes=1
  Vector Concatenate : Concatenate  NumInputs=3  Mode=Multidimensional array
  Vector Concatenate1 : Concatenate  NumInputs=3  Mode=Multidimensional array
  Vector Concatenate2 : Concatenate  NumInputs=3  Mode=Multidimensional array
  Out1 : Outport
  Out2 : Outport  Port=2
  Out3 : Outport  Port=3
  wires:
  Selector2/1 -> Vector Concatenate/3
  Vector Concatenate/1 -> Out1/1
  Selector8/1 -> Vector Concatenate2/3
  Selector4/1 -> Vector Concatenate1/2
  Selector6/1 -> Vector Concatenate2/1
  R_0/1 -> Reshape/1
  Reshape/1 -> Selector8/1, Selector7/1, Selector6/1, Selector5/1, Selector4/1, Selector3/1, Selector2/1, Selector1/1, Selector/1
  Selector/1 -> Vector Concatenate/1
  Selector5/1 -> Vector Concatenate1/3
  Selector7/1 -> Vector Concatenate2/2
  Vector Concatenate2/1 -> Out3/1
  Vector Concatenate1/1 -> Out2/1
  Selector1/1 -> Vector Concatenate/2
  Selector3/1 -> Vector Concatenate1/1

== system massbalancer/TNet/TBalances/Term2/X ==
  R-0 : Inport
  Ddot : Inport  Port=2
  s : Inport  Port=3
  Wb : Inport  Port=4
  Cross Product : matrix_library/Cross Product
  Cross Product1 : matrix_library/Cross Product
  Product : Product
  Output : Outport
  wires:
  Cross Product1/1 -> Output/1
  s/1 -> Product/1
  Ddot/1 -> Product/2
  Product/1 -> Cross Product/2
  Wb/1 -> Cross Product/1
  R-0/1 -> Cross Product1/1
  Cross Product/1 -> Cross Product1/2

== system massbalancer/TNet/TBalances/Term2/Y ==
  R0 : Inport
  ddot : Inport  Port=2
  s : Inport  Port=3
  Wb : Inport  Port=4
  Cross Product : matrix_library/Cross Product
  Cross Product1 : matrix_library/Cross Product
  Product : Product
  Output : Outport
  wires:
  s/1 -> Product/1
  Product/1 -> Cross Product/2
  R0/1 -> Cross Product1/1
  Cross Product/1 -> Cross Product1/2
  ddot/1 -> Product/2
  Wb/1 -> Cross Product/1
  Cross Product1/1 -> Output/1

== system massbalancer/TNet/TBalances/Term2/Z ==
  ddot : Inport
  R0 : Inport  Port=2
  s : Inport  Port=3
  Wb : Inport  Port=4
  Cross Product : matrix_library/Cross Product
  Cross Product1 : matrix_library/Cross Product
  Product : Product
  Output1 : Outport
  wires:
  s/1 -> Product/1
  Product/1 -> Cross Product/2
  R0/1 -> Cross Product1/1
  Cross Product/1 -> Cross Product1/2
  ddot/1 -> Product/2
  Wb/1 -> Cross Product/1
  Cross Product1/1 -> Output1/1

== system massbalancer/TNet/TBalances/Term3/Subsystem1 ==
  R_0 : Inport
  Reshape : Reshape  OutputDimensionality=Column vector (2-D)  OutputDimensions=[1,3]
  Selector : Selector  InputPortWidth=9  IndexOptions=Index vector (dialog)  Indices=[1]  OutputSizes=1
  Selector1 : Selector  InputPortWidth=9  IndexOptions=Index vector (dialog)  Indices=[2]  OutputSizes=1
  Selector2 : Selector  InputPortWidth=9  IndexOptions=Index vector (dialog)  Indices=[3]  OutputSizes=1
  Selector3 : Selector  InputPortWidth=9  IndexOptions=Index vector (dialog)  Indices=[4]  OutputSizes=1
  Selector4 : Selector  InputPortWidth=9  IndexOptions=Index vector (dialog)  Indices=[5]  OutputSizes=1
  Selector5 : Selector  InputPortWidth=9  IndexOptions=Index vector (dialog)  Indices=[6]  OutputSizes=1
  Selector6 : Selector  InputPortWidth=9  IndexOptions=Index vector (dialog)  Indices=[7]  OutputSizes=1
  Selector7 : Selector  InputPortWidth=9  IndexOptions=Index vector (dialog)  Indices=[8]  OutputSizes=1
  Selector8 : Selector  InputPortWidth=9  IndexOptions=Index vector (dialog)  Indices=[9]  OutputSizes=1
  Vector Concatenate : Concatenate  NumInputs=3  Mode=Multidimensional array
  Vector Concatenate1 : Concatenate  NumInputs=3  Mode=Multidimensional array
  Vector Concatenate2 : Concatenate  NumInputs=3  Mode=Multidimensional array
  Out1 : Outport
  Out2 : Outport  Port=2
  Out3 : Outport  Port=3
  wires:
  Selector3/1 -> Vector Concatenate1/1
  Selector1/1 -> Vector Concatenate/2
  Vector Concatenate1/1 -> Out2/1
  Vector Concatenate2/1 -> Out3/1
  Selector7/1 -> Vector Concatenate2/2
  Selector5/1 -> Vector Concatenate1/3
  Selector/1 -> Vector Concatenate/1
  Reshape/1 -> Selector/1, Selector1/1, Selector2/1, Selector3/1, Selector4/1, Selector5/1, Selector6/1, Selector7/1, Selector8/1
  R_0/1 -> Reshape/1
  Selector6/1 -> Vector Concatenate2/1
  Selector4/1 -> Vector Concatenate1/2
  Selector8/1 -> Vector Concatenate2/3
  Vector Concatenate/1 -> Out1/1
  Selector2/1 -> Vector Concatenate/3

== system massbalancer/TNet/TBalances/Term3/Subsystem3 ==
  R_0 : Inport
  Reshape : Reshape  OutputDimensionality=Column vector (2-D)  OutputDimensions=[1,3]
  Selector : Selector  InputPortWidth=9  IndexOptions=Index vector (dialog)  Indices=[1]  OutputSizes=1
  Selector1 : Selector  InputPortWidth=9  IndexOptions=Index vector (dialog)  Indices=[2]  OutputSizes=1
  Selector2 : Selector  InputPortWidth=9  IndexOptions=Index vector (dialog)  Indices=[3]  OutputSizes=1
  Selector3 : Selector  InputPortWidth=9  IndexOptions=Index vector (dialog)  Indices=[4]  OutputSizes=1
  Selector4 : Selector  InputPortWidth=9  IndexOptions=Index vector (dialog)  Indices=[5]  OutputSizes=1
  Selector5 : Selector  InputPortWidth=9  IndexOptions=Index vector (dialog)  Indices=[6]  OutputSizes=1
  Selector6 : Selector  InputPortWidth=9  IndexOptions=Index vector (dialog)  Indices=[7]  OutputSizes=1
  Selector7 : Selector  InputPortWidth=9  IndexOptions=Index vector (dialog)  Indices=[8]  OutputSizes=1
  Selector8 : Selector  InputPortWidth=9  IndexOptions=Index vector (dialog)  Indices=[9]  OutputSizes=1
  Vector Concatenate : Concatenate  NumInputs=3  Mode=Multidimensional array
  Vector Concatenate1 : Concatenate  NumInputs=3  Mode=Multidimensional array
  Vector Concatenate2 : Concatenate  NumInputs=3  Mode=Multidimensional array
  Out1 : Outport
  Out2 : Outport  Port=2
  Out3 : Outport  Port=3
  wires:
  Selector2/1 -> Vector Concatenate/3
  Vector Concatenate/1 -> Out1/1
  Selector8/1 -> Vector Concatenate2/3
  Selector4/1 -> Vector Concatenate1/2
  Selector6/1 -> Vector Concatenate2/1
  R_0/1 -> Reshape/1
  Reshape/1 -> Selector8/1, Selector7/1, Selector6/1, Selector5/1, Selector4/1, Selector3/1, Selector2/1, Selector1/1, Selector/1
  Selector/1 -> Vector Concatenate/1
  Selector5/1 -> Vector Concatenate1/3
  Selector7/1 -> Vector Concatenate2/2
  Vector Concatenate2/1 -> Out3/1
  Vector Concatenate1/1 -> Out2/1
  Selector1/1 -> Vector Concatenate/2
  Selector3/1 -> Vector Concatenate1/1

== system massbalancer/TNet/TBalances/Term3/X ==
  ddoubledot : Inport
  s : Inport  Port=2
  r : Inport  Port=3
  Cross Product : matrix_library/Cross Product
  Product : Product
  y : Outport
  wires:
  Cross Product/1 -> y/1
  ddoubledot/1 -> Product/1
  Product/1 -> Cross Product/2
  r/1 -> Cross Product/1
  s/1 -> Product/2

== system massbalancer/TNet/TBalances/Term3/Y ==
  ddoubledot : Inport
  s : Inport  Port=2
  r : Inport  Port=3
  Cross Product : matrix_library/Cross Product
  Product : Product
  y : Outport
  wires:
  Cross Product/1 -> y/1
  ddoubledot/1 -> Product/1
  Product/1 -> Cross Product/2
  r/1 -> Cross Product/1
  s/1 -> Product/2

== system massbalancer/TNet/TBalances/Term3/Z ==
  r : Inport
  s : Inport  Port=2
  ddoubledot : Inport  Port=3
  Cross Product : matrix_library/Cross Product
  Display : Display
  Product : Product
  y : Outport
  wires:
  Cross Product/1 -> Display/1, y/1
  ddoubledot/1 -> Product/1
  s/1 -> Product/2
  Product/1 -> Cross Product/2
  r/1 -> Cross Product/1
